simulink model "Controller"  (R2020b)
settings: Solver=ode15s  StartTime=0.0  StopTime=0.2  RelTol=1e-3
values from neighbouring files (symbols this model uses):
  Kd = 0.24162    [MotorPositiondData.sldd]
  Ki = 1902.7038    [MotorPositiondData.sldd]
  Kp = 44.5268    [MotorPositiondData.sldd]
  N = 2006.7432    [MotorPositiondData.sldd]
settings Model: DataDictionary=MotorPositiondData.sldd  Creator=Pavan  LastModifiedBy=Pavan
settings SolverCC: AlgebraicLoopSolver=LineSearch
settings DataIOCC: SaveOutput=off  SaveTime=off

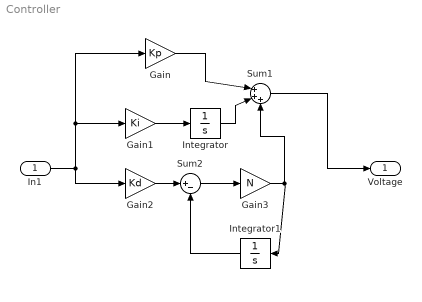
== system Controller ==
  In1 : Inport  OutDataTypeStr=double  PortDimensions=1  SampleTime=0
  Gain : Gain  Gain=Kp
  Gain1 : Gain  Gain=Ki
  Gain2 : Gain  Gain=Kd
  Gain3 : Gain  Gain=N
  Integrator : Integrator
  Integrator1 : Integrator
  Sum1 : Sum  Inputs=|+++
  Sum2 : Sum  Inputs=|+-
  Voltage : Outport  OutDataTypeStr=double  PortDimensions=1  SampleTime=0
  wires:
  In1/1 -> Gain/1, Gain1/1, Gain2/1
  Gain/1 -> Sum1/1
  Gain3/1 -> Integrator1/1, Sum1/3
  Integrator/1 -> Sum1/2
  Integrator1/1 -> Sum2/2
  Gain1/1 -> Integrator/1
  Sum2/1 -> Gain3/1
  Sum1/1 -> Voltage/1
  Gain2/1 -> Sum2/1
